simulink model "empezando"  (R2019a)
settings: Solver=VariableStepAuto  StartTime=0.0  StopTime=50  RelTol=1e-3
values from neighbouring files (symbols this model uses):
  alfa_cu = 3.9 * 10^(-3)    (= 0.0039)    [Datos.m]
  bl = 0    [Datos.m]
  bm = 1.5 * 10^(-5)    (= 1.5e-05)    [Datos.m]
  Cts = 0.818    [Datos.m]
  Id0 = 0.5    [Datos.m]    (also in punto6plot.m)
  Jl = 0.2520    (= 0.252)    [Datos.m]
  Jm = 3.1 * 10^(-6)    (= 3.1e-06)    [Datos.m]
  Kid = 0    [Datos.m]
  Kiq = 0    [Datos.m]
  lambda_m_r = 0.01546    [Datos.m]
  Ld = 6.6e-3    (= 0.0066)    [Datos.m]
  Lls = 0.8e-3    (= 0.0008)    [Datos.m]
  Lq = 5.8e-3    (= 0.0058)    [Datos.m]
  Pp = 3    [Datos.m]
  r = 314.3008    [Datos.m]
  Rts_amb = 146.7    [Datos.m]
undefined symbols (not defined in the file or in its folder): magnitude, sigbuilder_block
settings Model: Creator=lucastrubiano  LastModifiedBy=renzo

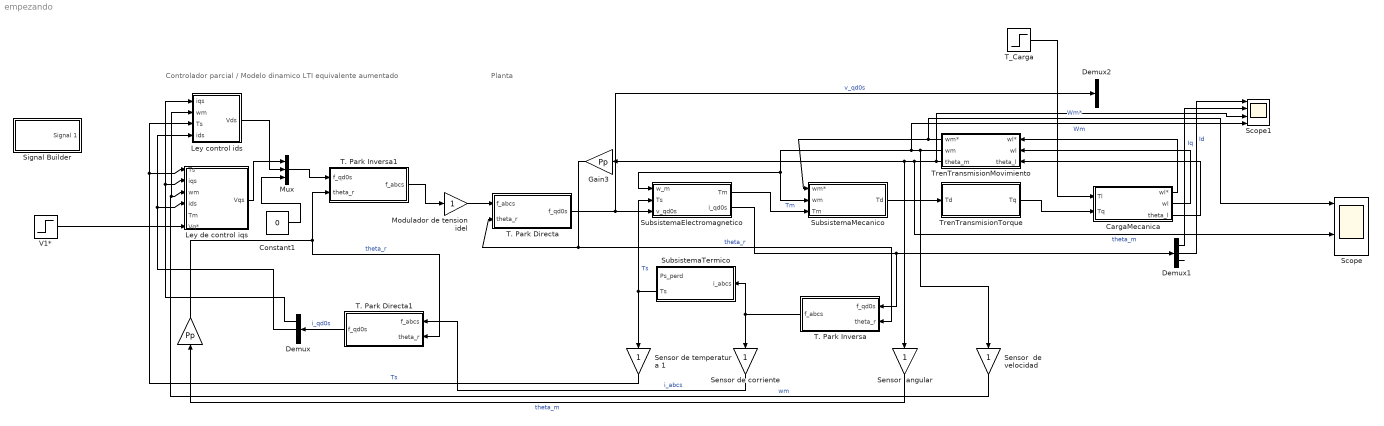
== system empezando ==
  note: Controlador parcial / Modelo dinamico LTI equivalente aumentado
  note: Planta
  " " : Gain  Gain=Pp
  CargaMecanica : Subsystem
  Constant1 : Constant  Value=0
  Demux : Demux  Outputs=3
  Demux1 : Demux  Outputs=3
  Demux2 : Demux  Outputs=3
  Gain3 : Gain  Gain=Pp
  Ley control ids : Subsystem
  Ley de control iqs : Subsystem
  "Modulador de tension idel " : Gain
  Mux : Mux  Inputs=3
  Scope : Scope  NumInputPorts=4
  Scope1 : Scope  NumInputPorts=4
  Sensor  angular : Gain
  Sensor  de velocidad : Gain
  "Sensor de corriente " : Gain
  Sensor de temperatura 1 : Gain
  Signal Builder : Subsystem  Tag=STV Subsys  LoadFcn=sigbuilder_block('load');  StartFcn=sigbuilder_block('start');  StopFcn=sigbuilder_block('stop');  ClipboardFcn=sigbuilder_block('clipboard');  mask(Sigbuilder block){tuvar=[0:10]}
      mask help: Simulink:masks:SigbuilderBlock_MD
      mask init:
      | if ~strcmp(get_param(bdroot(gcbh),'SimulationStatus'),'stopped') tuvar = sigbuilder_block('maskInit'); end
      settings: CopyFcn=sigbuilder_block('copy');  DeleteFcn=sigbuilder_block('delete');  ModelCloseFcn=sigbuilder_block('modelClose');  PreSaveFcn=sigbuilder_block('preSave');  PauseFcn=sigbuilder_block('pause');  ContinueFcn=sigbuilder_block('continue');  NameChangeFcn=sigbuilder_block('namechange');  OpenFcn=sigbuilder_block('open',[437.6 153 550.4 359.25 ]);  CloseFcn=sigbuilder_block('close');
      mask Display: plot(0, 0, 100, 100,[2, 2, 32, 32, 2], [68, 8, 8, 68, 68],[32, 2], [38, 38], [32, 19, 2],[53, 60, 44], [32, 17, 17, 2],[16, 16, 31, 31]);txt = getActiveGroup(gcbh);text(2, 100, txt,'verticalAlignment', 'top');
  SubsistemaElectromagnetico : Subsystem
  SubsistemaMecanico : Subsystem
  SubsistemaTermico : Subsystem
  T. Park Directa : Subsystem
  T. Park Directa1 : Subsystem
  T. Park Inversa : Subsystem
  T. Park Inversa1 : Subsystem
  T_Carga : Step  Time=5  After=0  SampleTime=0
  TrenTransmisionMovimiento : Subsystem
  TrenTransmisionTorque : Subsystem
  V1* : Step  After=10  SampleTime=0
  wires:
  CargaMecanica/1(wl*) -> TrenTransmisionMovimiento/1(wl*)
  CargaMecanica/2(wl) -> TrenTransmisionMovimiento/2(wl)
  CargaMecanica/3(theta_l) -> TrenTransmisionMovimiento/3(theta_l)
  T_Carga/1 -> CargaMecanica/1(Tl)
  SubsistemaElectromagnetico/1(Tm) -> SubsistemaMecanico/3(Tm)  "Tm"
  SubsistemaMecanico/1(Td) -> TrenTransmisionTorque/1(Td)
  TrenTransmisionMovimiento/1(wm*) -> Scope/1, SubsistemaMecanico/1(wm*)  "Wm*"
  TrenTransmisionMovimiento/2(wm) -> Sensor  de velocidad/1, Scope1/4, SubsistemaElectromagnetico/1(w_m), SubsistemaMecanico/2(wm)  "Wm"
  TrenTransmisionMovimiento/3(theta_m) -> Scope1/3, Scope/3, Sensor  angular/1, Gain3/1  "theta_m"
  SubsistemaElectromagnetico/2(i_qd0s) -> Demux1/1, T. Park Inversa/1(f_qd0s)
  SubsistemaTermico/2(Ts) -> SubsistemaElectromagnetico/2(Ts), Sensor de temperatura 1/1  "Ts"
  TrenTransmisionTorque/1(Tq) -> CargaMecanica/2(Tq)
  T. Park Directa/1(f_qd0s) -> Demux2/1, SubsistemaElectromagnetico/3("v_qd0s ")  "v_qd0s"
  Gain3/1 -> T. Park Directa/2(theta_r), T. Park Inversa/2(theta_r)  "theta_r"
  T. Park Inversa/1(f_abcs) -> "Sensor de corriente "/1, SubsistemaTermico/1(i_abcs)
  Sensor  angular/1 -> " "/1  "theta_m"
  " "/1 -> T. Park Inversa1/2(theta_r), T. Park Directa1/2(theta_r)  "theta_r"
  "Sensor de corriente "/1 -> T. Park Directa1/1(f_abcs)  "i_abcs"
  T. Park Directa1/1(f_qd0s) -> Demux/1  "i_qd0s"
  Sensor  de velocidad/1 -> Ley control ids/2(wm), Ley de control iqs/3(wm)  "wm"
  Sensor de temperatura 1/1 -> Ley control ids/3(Ts), Ley de control iqs/1(Ts)  "Ts"
  Demux/2 -> Ley control ids/4(ids), Ley de control iqs/4(ids)
  Demux/1 -> Ley control ids/1(iqs), Ley de control iqs/2(iqs)
  V1*/1 -> Ley de control iqs/6(Vq*)
  Constant1/1 -> Mux/3
  Mux/1 -> T. Park Inversa1/1(f_qd0s)
  T. Park Inversa1/1(f_abcs) -> "Modulador de tension idel "/1
  "Modulador de tension idel "/1 -> T. Park Directa/1(f_abcs)
  Ley control ids/1(Vds) -> Mux/2
  Ley de control iqs/1(Vqs) -> Mux/1
  Demux1/3 -> ?
  Demux1/1 -> Scope1/2  "Iq"
  Demux1/2 -> Scope1/1  "Id"

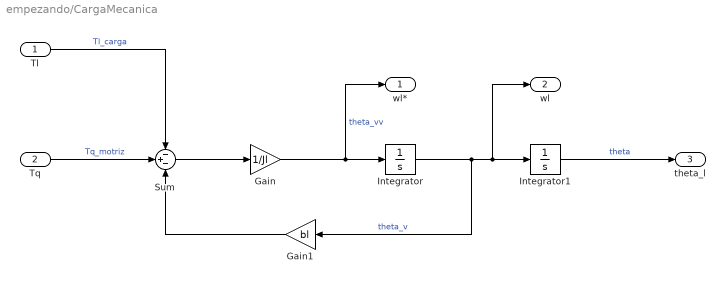
== system empezando/CargaMecanica ==
  Tl : Inport
  Tq : Inport  Port=2
  Gain : Gain  Gain=1/Jl
  Gain1 : Gain  Gain=bl
  Integrator : Integrator
  Integrator1 : Integrator
  Sum : Sum  Inputs=-+-
  wl* : Outport  VectorParamsAs1DForOutWhenUnconnected=on
  wl : Outport  Port=2  VectorParamsAs1DForOutWhenUnconnected=on
  theta_l : Outport  Port=3  VectorParamsAs1DForOutWhenUnconnected=on
  wires:
  Tq/1 -> Sum/2  "Tq_motriz"
  Sum/1 -> Gain/1
  Gain1/1 -> Sum/3
  Tl/1 -> Sum/1  "Tl_carga"
  Integrator/1 -> Gain1/1, wl/1, Integrator1/1  "theta_v"
  Integrator1/1 -> theta_l/1  "theta"
  Gain/1 -> wl*/1, Integrator/1  "theta_vv"

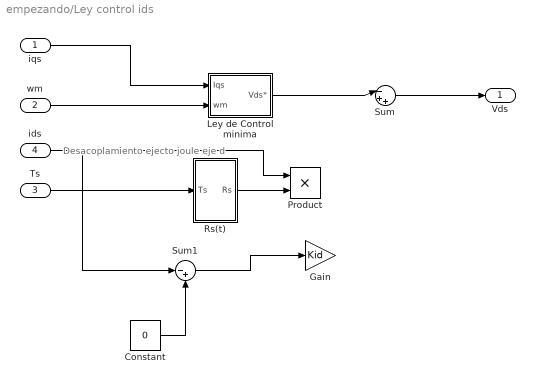
== system empezando/Ley control ids ==
  note: Desacoplamiento ejecto joule eje d
  iqs : Inport
  wm : Inport  Port=2
  Ts : Inport  Port=3
  ids : Inport  Port=4
  Constant : Constant  Value=0
  Gain : Gain  Gain=Kid
  Ley de Control minima : Subsystem
  Product : Product
  Rs(t) : Subsystem
  Sum : Sum  Inputs=|-++
  Sum1 : Sum  Inputs=|-+
  Vds : Outport
  wires:
  wm/1 -> Ley de Control minima/2(wm)
  iqs/1 -> Ley de Control minima/1(Iqs)
  Ley de Control minima/1(Vds*) -> Sum/1
  Rs(t)/1(Rs) -> Product/2
  Sum/1 -> Vds/1
  Ts/1 -> Rs(t)/1(Ts)
  ids/1 -> Sum1/1, Product/1
  Constant/1 -> Sum1/2
  Sum1/1 -> Gain/1

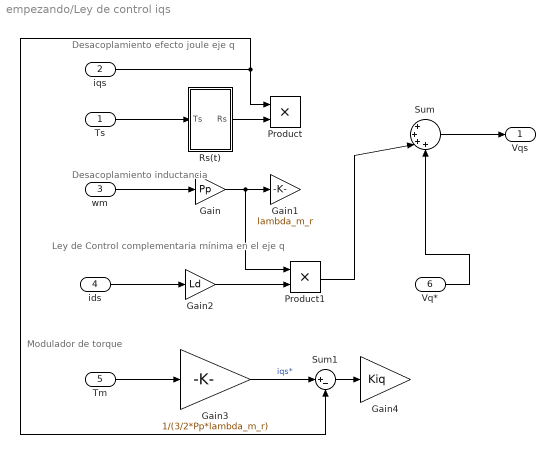
== system empezando/Ley de control iqs ==
  note: Desacoplamiento inductancia
  note: Desacoplamiento efecto joule eje q
  note: Modulador de torque
  note: Ley de Control complementaria mínima en el eje q
  Ts : Inport
  iqs : Inport  Port=2
  wm : Inport  Port=3
  ids : Inport  Port=4
  "Tm " : Inport  Port=5
  Vq* : Inport  Port=6
  Gain : Gain  Gain=Pp
  Gain1 : Gain  Gain=lambda_m_r
  Gain2 : Gain  Gain=Ld
  Gain3 : Gain  Gain=1/(3/2*Pp*lambda_m_r)
  Gain4 : Gain  Gain=Kiq
  Product : Product
  Product1 : Product
  Rs(t) : Subsystem
  Sum : Sum  Inputs=|++++
  Sum1 : Sum  Inputs=|+-
  Vqs : Outport
  wires:
  Rs(t)/1(Rs) -> Product/2
  Ts/1 -> Rs(t)/1(Ts)
  iqs/1 -> Sum1/2, Product/1
  wm/1 -> Gain/1
  Gain/1 -> Product1/1, Gain1/1
  ids/1 -> Gain2/1
  Gain2/1 -> Product1/2
  Product1/1 -> Sum/3
  Sum/1 -> Vqs/1
  "Tm "/1 -> Gain3/1
  Gain3/1 -> Sum1/1  "iqs*"
  Sum1/1 -> Gain4/1
  Vq*/1 -> Sum/4

== system empezando/Signal Builder ==
  Demux : Demux  Tag=STV Demux  Outputs=1
  FromWs : FromWorkspace  Tag=STV FromWs  VariableName=tuvar  SampleTime=0
      SigBuilderData=|
      | common.afterFinalStr = 'Extrapolate'
      | common.sampleTime = 0
      | dataSet.timeRange = [0 10]
      | dataSet.name = 'Group 1'
      | sbobj.Groups.Name = 'Group 1'
      | sbobj.Groups.Signals.Name = 'Signal 1'
      | sbobj.Groups.Signals.XData = [0 4 6 10]
      | sbobj.Groups.Signals.YData = [-0.005 0.04 1 1.005]
  Signal 1 : Outport  Tag=STV Outport
  wires:
  Demux/1 -> Signal 1/1
  FromWs/1 -> Demux/1

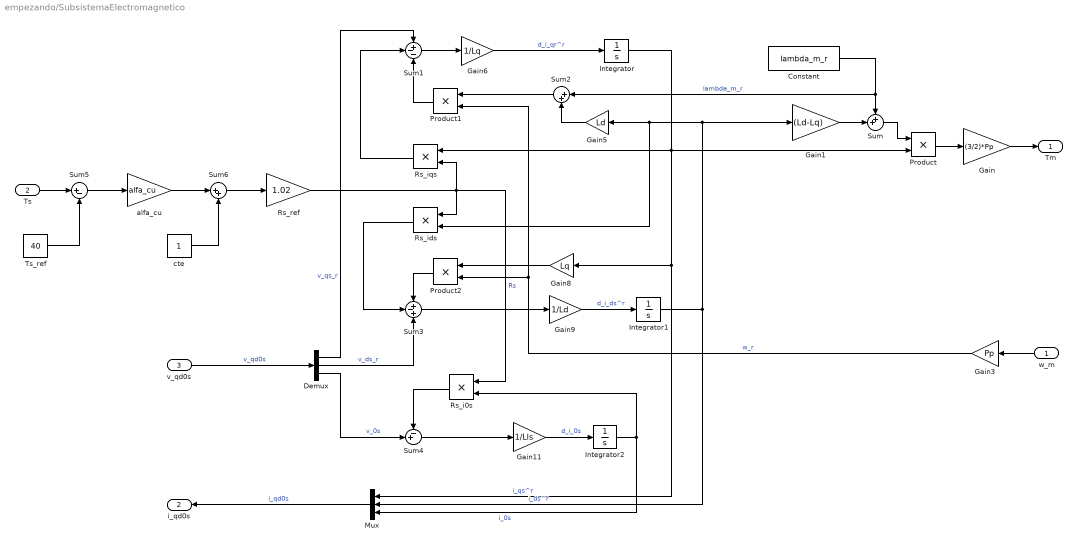
== system empezando/SubsistemaElectromagnetico ==
  w_m : Inport
  Ts : Inport  Port=2
  "v_qd0s " : Inport  Port=3
  Constant : Constant  Value=lambda_m_r
  Demux : Demux  Outputs=3
  Gain : Gain  Gain=(3/2)*Pp
  Gain1 : Gain  Gain=(Ld-Lq)
  Gain11 : Gain  Gain=1/Lls
  Gain3 : Gain  Gain=Pp
  Gain5 : Gain  Gain=Ld
  Gain6 : Gain  Gain=1/Lq
  Gain8 : Gain  Gain=Lq
  Gain9 : Gain  Gain=1/Ld
  Integrator : Integrator
  Integrator1 : Integrator  InitialCondition=Id0
  Integrator2 : Integrator
  Mux : Mux  Inputs=3
  Product : Product
  Product1 : Product
  Product2 : Product
  Rs_i0s : Product
  Rs_ids : Product
  Rs_iqs : Product
  Rs_ref : Gain  Gain=1.02
  Sum : Sum  Inputs=++|
  Sum1 : Sum  Inputs=+--
  Sum2 : Sum  Inputs=|++
  Sum3 : Sum  Inputs=+-+
  Sum4 : Sum  Inputs=-+|
  Sum5 : Sum  Inputs=|+-
  Sum6 : Sum  Inputs=|++
  Ts_ref : Constant  Value=40
  alfa_cu : Gain  Gain=alfa_cu
  cte : Constant
  Tm : Outport  VectorParamsAs1DForOutWhenUnconnected=on
  i_qd0s : Outport  Port=2  VectorParamsAs1DForOutWhenUnconnected=on
  wires:
  Gain/1 -> Tm/1
  Product/1 -> Gain/1
  Integrator/1 -> Mux/1, Gain8/1, Product/2, Rs_iqs/1  "i_qs^r"
  Sum/1 -> Product/1
  Gain1/1 -> Sum/2
  Integrator1/1 -> Gain5/1, Rs_ids/2, Gain1/1, Mux/2  "i_ds^r"
  Constant/1 -> Sum2/1, Sum/1  "lambda_m_r"
  w_m/1 -> Gain3/1
  "v_qd0s "/1 -> Demux/1  "v_qd0s"
  Demux/1 -> Sum1/1  "v_qs_r"
  Demux/2 -> Sum3/3  "v_ds_r"
  Demux/3 -> Sum4/2  "v_0s"
  Rs_iqs/1 -> Sum1/2
  Product1/1 -> Sum1/3
  Gain3/1 -> Product1/2, Product2/2  "w_r"
  Sum2/1 -> Product1/1
  Gain5/1 -> Sum2/2
  Sum1/1 -> Gain6/1
  Gain6/1 -> Integrator/1  "d_i_qr^r"
  Rs_ids/1 -> Sum3/2
  Product2/1 -> Sum3/1
  Gain8/1 -> Product2/1
  Sum3/1 -> Gain9/1
  Gain9/1 -> Integrator1/1  "d_i_ds^r"
  Rs_i0s/1 -> Sum4/1
  Integrator2/1 -> Rs_i0s/2, Mux/3  "i_0s"
  Sum4/1 -> Gain11/1
  Gain11/1 -> Integrator2/1  "d_i_0s"
  Mux/1 -> i_qd0s/1  "i_qd0s"
  Ts/1 -> Sum5/1
  Ts_ref/1 -> Sum5/2
  Sum5/1 -> alfa_cu/1
  alfa_cu/1 -> Sum6/1
  cte/1 -> Sum6/2
  Sum6/1 -> Rs_ref/1
  Rs_ref/1 -> Rs_ids/1, Rs_i0s/1, Rs_iqs/2  "Rs"

== system empezando/SubsistemaMecanico ==
  wm* : Inport
  wm : Inport  Port=2
  Tm : Inport  Port=3
  Gain1 : Gain  Gain=bm
  Gain2 : Gain  Gain=Jm
  Sum : Sum  Inputs=--+
  Td : Outport  VectorParamsAs1DForOutWhenUnconnected=on
  wires:
  wm*/1 -> Gain2/1
  wm/1 -> Gain1/1
  Gain2/1 -> Sum/1
  Gain1/1 -> Sum/2
  Sum/1 -> Td/1
  Tm/1 -> Sum/3

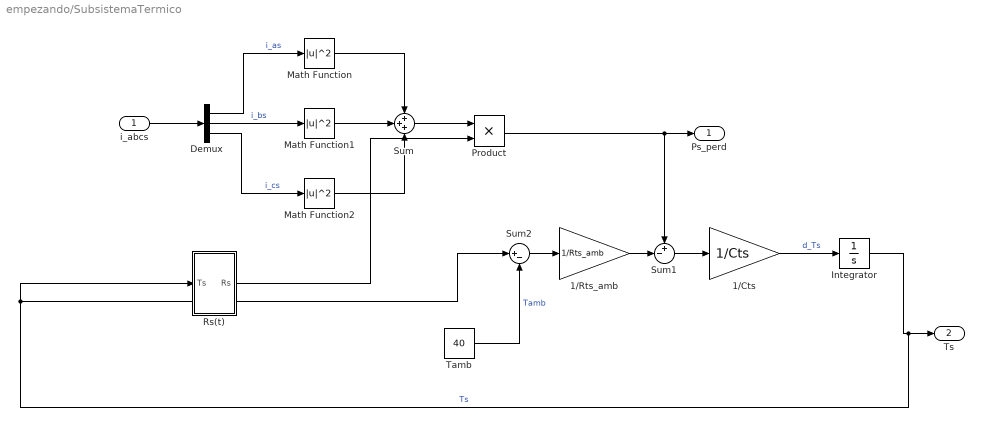
== system empezando/SubsistemaTermico ==
  i_abcs : Inport
  1/Cts : Gain  Gain=1/Cts
  1/Rts_amb : Gain  Gain=1/Rts_amb
  Demux : Demux  Outputs=3
  Integrator : Integrator
  Math Function : Math  Operator=magnitude^2  SaturateOnIntegerOverflow=on
  Math Function1 : Math  Operator=magnitude^2  SaturateOnIntegerOverflow=on
  Math Function2 : Math  Operator=magnitude^2  SaturateOnIntegerOverflow=on
  Product : Product
  Rs(t) : Subsystem
  Sum : Sum  Inputs=3
  Sum1 : Sum  Inputs=+-|
  Sum2 : Sum  Inputs=|+-
  Tamb : Constant  Value=40
  Ps_perd : Outport  VectorParamsAs1DForOutWhenUnconnected=on
  Ts : Outport  Port=2  VectorParamsAs1DForOutWhenUnconnected=on
  wires:
  i_abcs/1 -> Demux/1
  Demux/1 -> Math Function/1  "i_as"
  Demux/2 -> Math Function1/1  "i_bs"
  Demux/3 -> Math Function2/1  "i_cs"
  Math Function1/1 -> Sum/2
  Math Function/1 -> Sum/1
  Math Function2/1 -> Sum/3
  Sum/1 -> Product/1
  Product/1 -> Sum1/1, Ps_perd/1
  Tamb/1 -> Sum2/2  "Tamb"
  Sum2/1 -> 1/Rts_amb/1
  1/Rts_amb/1 -> Sum1/2
  Sum1/1 -> 1/Cts/1
  1/Cts/1 -> Integrator/1  "d_Ts"
  Integrator/1 -> Rs(t)/1(Ts), Sum2/1, Ts/1  "Ts"
  Rs(t)/1(Rs) -> Product/2

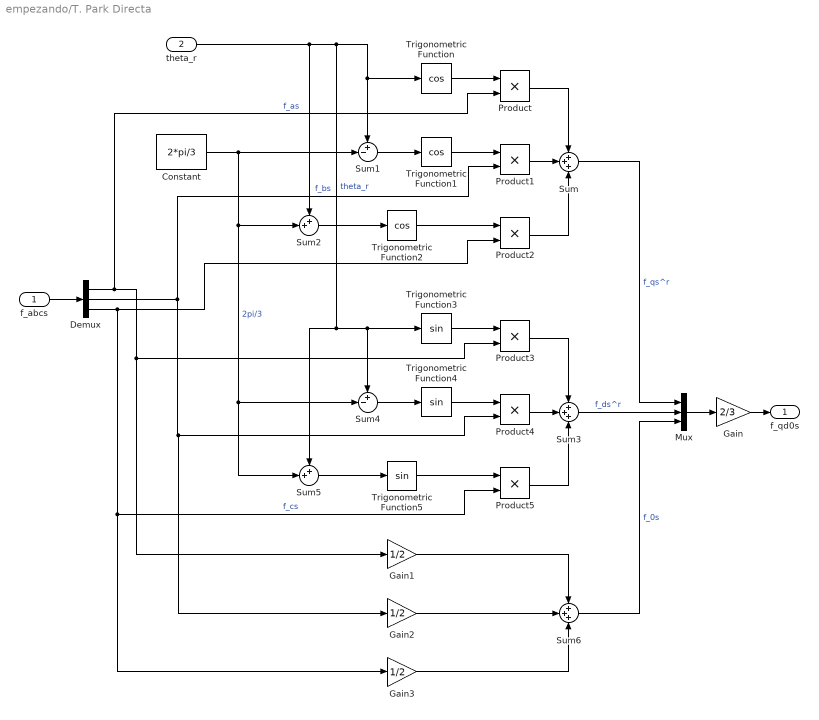
== system empezando/T. Park Directa ==
  f_abcs : Inport
  theta_r : Inport  Port=2
  Constant : Constant  Value=2*pi/3
  Demux : Demux  Outputs=3
  Gain : Gain  Gain=2/3
  Gain1 : Gain  Gain=1/2
  Gain2 : Gain  Gain=1/2
  Gain3 : Gain  Gain=1/2
  Mux : Mux  Inputs=3
  Product{,1..5} (6 alike) : Product
  Sum : Sum  Inputs=3
  Sum1 : Sum  Inputs=+-|
  Sum2 : Sum  Inputs=++|
  Sum3 : Sum  Inputs=3
  Sum4 : Sum  Inputs=+-|
  Sum5 : Sum  Inputs=++|
  Sum6 : Sum  Inputs=3
  Trigonometric Function : Trigonometry  Operator=cos
  Trigonometric Function1 : Trigonometry  Operator=cos
  Trigonometric Function2 : Trigonometry  Operator=cos
  Trigonometric Function3 : Trigonometry
  Trigonometric Function4 : Trigonometry
  Trigonometric Function5 : Trigonometry
  f_qd0s : Outport  VectorParamsAs1DForOutWhenUnconnected=on
  wires:
  Mux/1 -> Gain/1
  f_abcs/1 -> Demux/1
  Demux/1 -> Gain1/1, Product3/2, Product/2  "f_as"
  Demux/2 -> Gain2/1, Product4/2, Product1/2  "f_bs"
  Demux/3 -> Gain3/1, Product5/2, Product2/2  "f_cs"
  Sum/1 -> Mux/1  "f_qs^r"
  Gain/1 -> f_qd0s/1
  Trigonometric Function/1 -> Product/1
  Product/1 -> Sum/1
  Sum1/1 -> Trigonometric Function1/1
  Constant/1 -> Sum5/2, Sum4/2, Sum2/2, Sum1/2  "2pi/3"
  Trigonometric Function1/1 -> Product1/1
  Product1/1 -> Sum/2
  Product2/1 -> Sum/3
  Trigonometric Function2/1 -> Product2/1
  Sum2/1 -> Trigonometric Function2/1
  Product4/1 -> Sum3/2
  Trigonometric Function5/1 -> Product5/1
  Sum5/1 -> Trigonometric Function5/1
  Product5/1 -> Sum3/3
  Product3/1 -> Sum3/1
  Trigonometric Function4/1 -> Product4/1
  Sum4/1 -> Trigonometric Function4/1
  Sum3/1 -> Mux/2  "f_ds^r"
  Trigonometric Function3/1 -> Product3/1
  theta_r/1 -> Sum5/1, Sum4/1, Trigonometric Function3/1, Trigonometric Function/1, Sum1/1, Sum2/1  "theta_r"
  Sum6/1 -> Mux/3  "f_0s"
  Gain3/1 -> Sum6/3
  Gain1/1 -> Sum6/1
  Gain2/1 -> Sum6/2

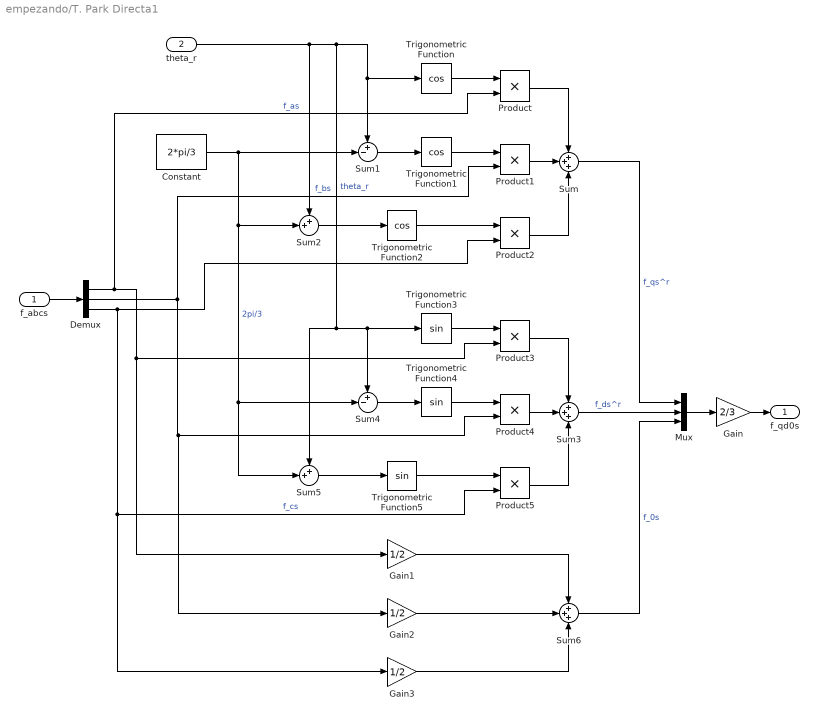
== system empezando/T. Park Directa1 ==
  f_abcs : Inport
  theta_r : Inport  Port=2
  Constant : Constant  Value=2*pi/3
  Demux : Demux  Outputs=3
  Gain : Gain  Gain=2/3
  Gain1 : Gain  Gain=1/2
  Gain2 : Gain  Gain=1/2
  Gain3 : Gain  Gain=1/2
  Mux : Mux  Inputs=3
  Product{,1..5} (6 alike) : Product
  Sum : Sum  Inputs=3
  Sum1 : Sum  Inputs=+-|
  Sum2 : Sum  Inputs=++|
  Sum3 : Sum  Inputs=3
  Sum4 : Sum  Inputs=+-|
  Sum5 : Sum  Inputs=++|
  Sum6 : Sum  Inputs=3
  Trigonometric Function : Trigonometry  Operator=cos
  Trigonometric Function1 : Trigonometry  Operator=cos
  Trigonometric Function2 : Trigonometry  Operator=cos
  Trigonometric Function3 : Trigonometry
  Trigonometric Function4 : Trigonometry
  Trigonometric Function5 : Trigonometry
  f_qd0s : Outport  VectorParamsAs1DForOutWhenUnconnected=on
  wires:
  Mux/1 -> Gain/1
  f_abcs/1 -> Demux/1
  Demux/1 -> Gain1/1, Product3/2, Product/2  "f_as"
  Demux/2 -> Gain2/1, Product4/2, Product1/2  "f_bs"
  Demux/3 -> Gain3/1, Product5/2, Product2/2  "f_cs"
  Sum/1 -> Mux/1  "f_qs^r"
  Gain/1 -> f_qd0s/1
  Trigonometric Function/1 -> Product/1
  Product/1 -> Sum/1
  Sum1/1 -> Trigonometric Function1/1
  Constant/1 -> Sum5/2, Sum4/2, Sum2/2, Sum1/2  "2pi/3"
  Trigonometric Function1/1 -> Product1/1
  Product1/1 -> Sum/2
  Product2/1 -> Sum/3
  Trigonometric Function2/1 -> Product2/1
  Sum2/1 -> Trigonometric Function2/1
  Product4/1 -> Sum3/2
  Trigonometric Function5/1 -> Product5/1
  Sum5/1 -> Trigonometric Function5/1
  Product5/1 -> Sum3/3
  Product3/1 -> Sum3/1
  Trigonometric Function4/1 -> Product4/1
  Sum4/1 -> Trigonometric Function4/1
  Sum3/1 -> Mux/2  "f_ds^r"
  Trigonometric Function3/1 -> Product3/1
  theta_r/1 -> Sum5/1, Sum4/1, Trigonometric Function3/1, Trigonometric Function/1, Sum1/1, Sum2/1  "theta_r"
  Sum6/1 -> Mux/3  "f_0s"
  Gain3/1 -> Sum6/3
  Gain1/1 -> Sum6/1
  Gain2/1 -> Sum6/2

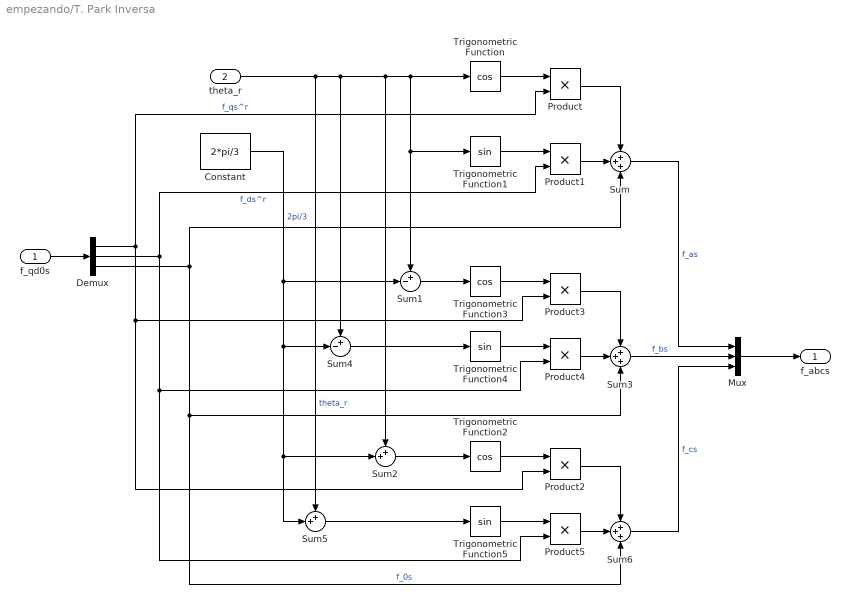
== system empezando/T. Park Inversa ==
  f_qd0s : Inport
  theta_r : Inport  Port=2
  Constant : Constant  Value=2*pi/3
  Demux : Demux  Outputs=3
  Mux : Mux  Inputs=3
  Product{,1..5} (6 alike) : Product
  Sum : Sum  Inputs=3
  Sum1 : Sum  Inputs=+-|
  Sum2 : Sum  Inputs=++|
  Sum3 : Sum  Inputs=3
  Sum4 : Sum  Inputs=+-|
  Sum5 : Sum  Inputs=++|
  Sum6 : Sum  Inputs=3
  Trigonometric Function : Trigonometry  Operator=cos
  Trigonometric Function1 : Trigonometry
  Trigonometric Function2 : Trigonometry  Operator=cos
  Trigonometric Function3 : Trigonometry  Operator=cos
  Trigonometric Function4 : Trigonometry
  Trigonometric Function5 : Trigonometry
  f_abcs : Outport  VectorParamsAs1DForOutWhenUnconnected=on
  wires:
  Trigonometric Function4/1 -> Product4/1
  f_qd0s/1 -> Demux/1
  Trigonometric Function/1 -> Product/1
  Constant/1 -> Sum1/2, Sum4/2, Sum2/2, Sum5/2  "2pi/3"
  Product1/1 -> Sum/2
  Mux/1 -> f_abcs/1
  Sum6/1 -> Mux/3  "f_cs"
  Product/1 -> Sum/1
  theta_r/1 -> Trigonometric Function/1, Trigonometric Function1/1, Sum1/1, Sum2/1, Sum4/1, Sum5/1  "theta_r"
  Product4/1 -> Sum3/2
  Sum3/1 -> Mux/2  "f_bs"
  Trigonometric Function1/1 -> Product1/1
  Sum/1 -> Mux/1  "f_as"
  Trigonometric Function3/1 -> Product3/1
  Product3/1 -> Sum3/1
  Sum4/1 -> Trigonometric Function4/1
  Demux/1 -> Product2/2, Product3/2, Product/2  "f_qs^r"
  Demux/2 -> Product5/2, Product4/2, Product1/2  "f_ds^r"
  Demux/3 -> Sum/3, Sum6/3, Sum3/3  "f_0s"
  Sum1/1 -> Trigonometric Function3/1
  Sum5/1 -> Trigonometric Function5/1
  Trigonometric Function5/1 -> Product5/1
  Trigonometric Function2/1 -> Product2/1
  Product2/1 -> Sum6/1
  Product5/1 -> Sum6/2
  Sum2/1 -> Trigonometric Function2/1

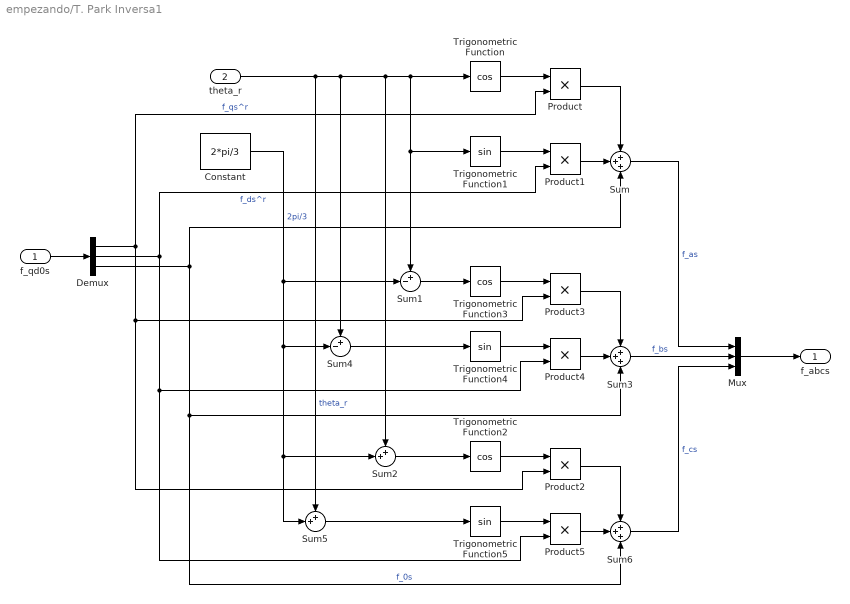
== system empezando/T. Park Inversa1 ==
  f_qd0s : Inport
  theta_r : Inport  Port=2
  Constant : Constant  Value=2*pi/3
  Demux : Demux  Outputs=3
  Mux : Mux  Inputs=3
  Product{,1..5} (6 alike) : Product
  Sum : Sum  Inputs=3
  Sum1 : Sum  Inputs=+-|
  Sum2 : Sum  Inputs=++|
  Sum3 : Sum  Inputs=3
  Sum4 : Sum  Inputs=+-|
  Sum5 : Sum  Inputs=++|
  Sum6 : Sum  Inputs=3
  Trigonometric Function : Trigonometry  Operator=cos
  Trigonometric Function1 : Trigonometry
  Trigonometric Function2 : Trigonometry  Operator=cos
  Trigonometric Function3 : Trigonometry  Operator=cos
  Trigonometric Function4 : Trigonometry
  Trigonometric Function5 : Trigonometry
  f_abcs : Outport  VectorParamsAs1DForOutWhenUnconnected=on
  wires:
  Trigonometric Function4/1 -> Product4/1
  f_qd0s/1 -> Demux/1
  Trigonometric Function/1 -> Product/1
  Constant/1 -> Sum1/2, Sum4/2, Sum2/2, Sum5/2  "2pi/3"
  Product1/1 -> Sum/2
  Mux/1 -> f_abcs/1
  Sum6/1 -> Mux/3  "f_cs"
  Product/1 -> Sum/1
  theta_r/1 -> Trigonometric Function/1, Trigonometric Function1/1, Sum1/1, Sum2/1, Sum4/1, Sum5/1  "theta_r"
  Product4/1 -> Sum3/2
  Sum3/1 -> Mux/2  "f_bs"
  Trigonometric Function1/1 -> Product1/1
  Sum/1 -> Mux/1  "f_as"
  Trigonometric Function3/1 -> Product3/1
  Product3/1 -> Sum3/1
  Sum4/1 -> Trigonometric Function4/1
  Demux/1 -> Product2/2, Product3/2, Product/2  "f_qs^r"
  Demux/2 -> Product5/2, Product4/2, Product1/2  "f_ds^r"
  Demux/3 -> Sum/3, Sum6/3, Sum3/3  "f_0s"
  Sum1/1 -> Trigonometric Function3/1
  Sum5/1 -> Trigonometric Function5/1
  Trigonometric Function5/1 -> Product5/1
  Trigonometric Function2/1 -> Product2/1
  Product2/1 -> Sum6/1
  Product5/1 -> Sum6/2
  Sum2/1 -> Trigonometric Function2/1

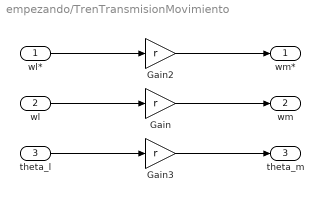
== system empezando/TrenTransmisionMovimiento ==
  wl* : Inport
  wl : Inport  Port=2
  theta_l : Inport  Port=3
  Gain : Gain  Gain=r
  Gain2 : Gain  Gain=r
  Gain3 : Gain  Gain=r
  wm* : Outport  VectorParamsAs1DForOutWhenUnconnected=on
  wm : Outport  Port=2  VectorParamsAs1DForOutWhenUnconnected=on
  theta_m : Outport  Port=3  VectorParamsAs1DForOutWhenUnconnected=on
  wires:
  Gain2/1 -> wm*/1
  wl/1 -> Gain/1
  wl*/1 -> Gain2/1
  Gain/1 -> wm/1
  theta_l/1 -> Gain3/1
  Gain3/1 -> theta_m/1

== system empezando/TrenTransmisionTorque ==
  Td : Inport
  Gain1 : Gain  Gain=r
  Tq : Outport  VectorParamsAs1DForOutWhenUnconnected=on
  wires:
  Td/1 -> Gain1/1
  Gain1/1 -> Tq/1

== system empezando/Ley control ids/Ley de Control minima ==
  Iqs : Inport
  wm : Inport  Port=2
  " 1" : Gain  Gain=Lq
  " 2" : Gain  Gain=Pp
  Product : Product
  Vds* : Outport
  wires:
  Iqs/1 -> " 1"/1  "iqs"
  " 1"/1 -> " 2"/1
  " 2"/1 -> Product/2
  wm/1 -> Product/1  "iqs"
  Product/1 -> Vds*/1

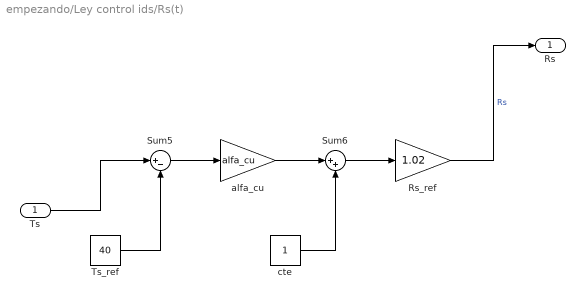
== system empezando/Ley control ids/Rs(t) ==
  Ts : Inport
  Rs_ref : Gain  Gain=1.02
  Sum5 : Sum  Inputs=|+-
  Sum6 : Sum  Inputs=|++
  Ts_ref : Constant  Value=40
  alfa_cu : Gain  Gain=alfa_cu
  cte : Constant
  Rs : Outport
  wires:
  alfa_cu/1 -> Sum6/1
  Sum6/1 -> Rs_ref/1
  Rs_ref/1 -> Rs/1  "Rs"
  Ts_ref/1 -> Sum5/2
  cte/1 -> Sum6/2
  Ts/1 -> Sum5/1
  Sum5/1 -> alfa_cu/1

== system empezando/Ley de control iqs/Rs(t) ==
  Ts : Inport
  Rs_ref : Gain  Gain=1.02
  Sum5 : Sum  Inputs=|+-
  Sum6 : Sum  Inputs=|++
  Ts_ref : Constant  Value=40
  alfa_cu : Gain  Gain=alfa_cu
  cte : Constant
  Rs : Outport
  wires:
  alfa_cu/1 -> Sum6/1
  Sum6/1 -> Rs_ref/1
  Rs_ref/1 -> Rs/1  "Rs"
  Ts_ref/1 -> Sum5/2
  cte/1 -> Sum6/2
  Ts/1 -> Sum5/1
  Sum5/1 -> alfa_cu/1

== system empezando/SubsistemaTermico/Rs(t) ==
  Ts : Inport
  Rs_ref : Gain  Gain=1.02
  Sum5 : Sum  Inputs=|+-
  Sum6 : Sum  Inputs=|++
  Ts_ref : Constant  Value=40
  alfa_cu : Gain  Gain=alfa_cu
  cte : Constant
  Rs : Outport
  wires:
  alfa_cu/1 -> Sum6/1
  Sum6/1 -> Rs_ref/1
  Rs_ref/1 -> Rs/1  "Rs"
  Ts_ref/1 -> Sum5/2
  cte/1 -> Sum6/2
  Ts/1 -> Sum5/1
  Sum5/1 -> alfa_cu/1
